simulink model "RollAngleHoldControlS"  (R2018b)
settings: Solver=VariableStepAuto  StartTime=0.0  StopTime=10.0  RelTol=1e-3
libraries: simulink x1
settings Model: Creator=cdjsd  LastModifiedBy=cdjsd

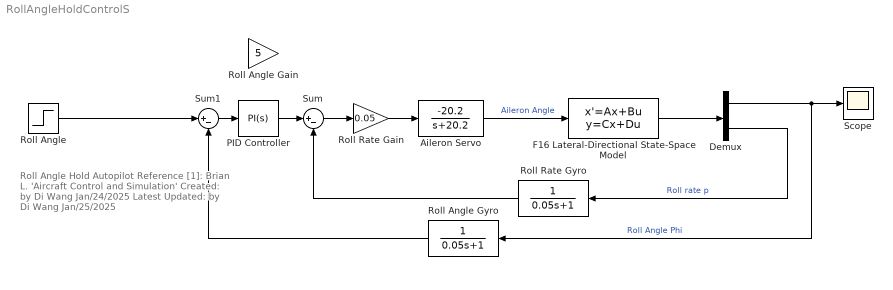
== system RollAngleHoldControlS ==
  note: Roll Angle Hold Autopilot
      | Reference [1]: Brian L. 'Aircraft Control and Simulation'
      | Created: by Di Wang Jan/24/2025
      | Latest Updated: by Di Wang Jan/25/2025
  Aileron Servo : TransferFcn  Numerator=[-20.2]  Denominator=[1 20.2]
  Demux : Demux  Outputs=2
  F16 Lateral-Directional State-Space Model : StateSpace  A=|  B=[2.9506e-4; 0; -7.3331e-1; -3.1865e-2]  C=|  D=zeros(2,1)  InitialCondition=0
      A=|
      | [-3.2201e-1 6.404e-2 3.6382e-2 -9.9167e-1;
      |      0 0 1 3.6928e-2;
      |      -30.649 0 -3.6784 6.6461e-1;
      |      8.5395 0 -2.5435e-2 -4.7637]
      C=|
      | [0 57.296 0 0;
      |      0 0 57.296 0]
  PID Controller : simulink/Continuous/PID Controller  Controller=PI  Form=Parallel  TimeDomain=Continuous-time  SampleTime=-1  IntegratorMethod=Forward Euler  FilterMethod=Forward Euler  ControllerParametersSource=internal  P=5  I=1  D=0  UseFilter=on  N=100  TunerSelectOption=Transfer Function Based (PID Tuner App)  InitialConditionSource=internal  InitialConditionForIntegrator=0  InitialConditionForFilter=0  DifferentiatorICPrevScaledInput=0  ExternalReset=none  TrackingMode=off  Kt=1  LimitOutput=off  UpperSaturationLimit=inf  LowerSaturationLimit=-inf  LinearizeAsGain=on  AntiWindupMode=none  Kb=1  POutMin=[]  POutMax=[]  IOutMin=[]  IOutMax=[]  DOutMin=[]  DOutMax=[]  NOutMin=[]  NOutMax=[]  SumOutMin=[]  SumOutMax=[]  SaturationOutMin=[]  SaturationOutMax=[]  PParamMin=[]  PParamMax=[]  IParamMin=[]  IParamMax=[]  DParamMin=[]  DParamMax=[]  NParamMin=[]  NParamMax=[]  KbParamMin=[]  KbParamMax=[]  KtParamMin=[]  KtParamMax=[]  KbOutMin=[]  KbOutMax=[]  KtOutMin=[]  KtOutMax=[]  IntegratorOutMin=[]  IntegratorOutMax=[]  FilterOutMin=[]  FilterOutMax=[]  SumI1OutMin=[]  SumI1OutMax=[]  SumI2OutMin=[]  SumI2OutMax=[]  SumI3OutMin=[]  SumI3OutMax=[]  SumI4OutMin=[]  SumI4OutMax=[]  SumDOutMin=[]  SumDOutMax=[]  DifferentiatorOutMin=[]  DifferentiatorOutMax=[]  FilterDiffOutCoefMin=[]  FilterDiffOutCoefMax=[]  ReciprocalOutMin=[]  ReciprocalOutMax=[]  SumDenOutMin=[]  SumDenOutMax=[]  SumNumOutMin=[]  SumNumOutMax=[]  DivideOutMin=[]  DivideOutMax=[]  IntegratorContinuousStateAttributes=''  IntegratorStateMustResolveToSignalObject=off  IntegratorRTWStateStorageClass=Auto  FilterContinuousStateAttributes=''  FilterStateMustResolveToSignalObject=off  FilterRTWStateStorageClass=Auto  ParallelPVariant=InternalParameters  IdealPVariant=Disabled  IVariant=InternalParameters  DVariant=Disabled  IntegratorVariant=Continuous  SatVariant=Disabled  AWVariant=Passthrough  PCopyVariant=Disabled  TRVariant=Disabled  FdbkBlocksVariant=Forward  IdealPFdbkVariant=Disabled  SatFdbkVariant=Disabled  DerivativeFilterVariant=Disabled  NVariant=Disabled  NCopyVariant=Disabled_SignalSpec  FilterICVariant=Disabled  IntegratorICVariant=InternalICs  ExternalResetVariant=Disabled  TRSumVariant=Passthrough  SumFdbkVariant=Disabled  SumVariant=Sum_PI
  Roll Angle : Step  SampleTime=0
  Roll Angle Gain : Gain  Gain=5
  Roll Angle Gyro : TransferFcn  Denominator=[0.05 1]
  Roll Rate Gain : Gain  Gain=0.05
  Roll Rate Gyro : TransferFcn  Denominator=[0.05 1]
  Scope : Scope
  Sum : Sum  Inputs=|+-
  Sum1 : Sum  Inputs=|+-
  wires:
  Aileron Servo/1 -> F16 Lateral-Directional State-Space Model/1  "Aileron Angle"
  F16 Lateral-Directional State-Space Model/1 -> Demux/1
  Roll Rate Gain/1 -> Aileron Servo/1
  Demux/2 -> Roll Rate Gyro/1  "Roll rate p"
  Demux/1 -> Roll Angle Gyro/1, Scope/1  "Roll Angle Phi"
  Sum/1 -> Roll Rate Gain/1
  Roll Rate Gyro/1 -> Sum/2
  PID Controller/1 -> Sum/1
  Sum1/1 -> PID Controller/1
  Roll Angle Gyro/1 -> Sum1/2
  Roll Angle/1 -> Sum1/1
